simulink model "pendulam"  (R2019a)
settings: Solver=VariableStepAuto  StartTime=0.0  StopTime=10  FixedStep=0.01  MaxStep=0.05  MinStep=0.001  RelTol=1e-3
undefined symbols (not defined in the file): sigbuilder_block
settings Model: Creator=HPP  LastModifiedBy=vardhah
settings SolverCC: InitialStep=0.01
settings DebuggingCC: UnderSpecifiedDimensionMsg=warning

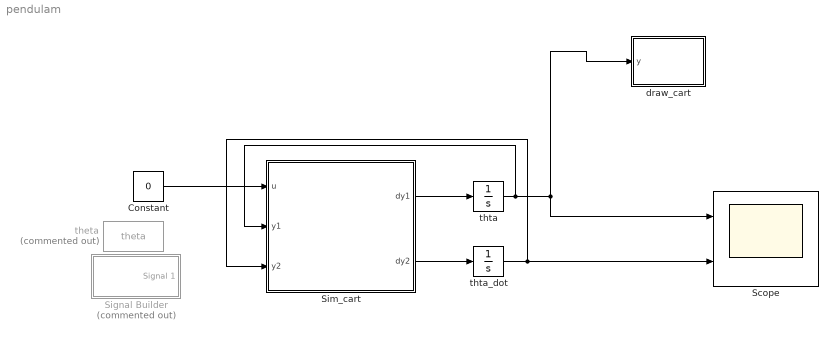
== system pendulam ==
  Constant : Constant  Value=0
  Scope : Scope  NumInputPorts=2
  Signal Builder : Subsystem  Tag=STV Subsys  Commented=on  LoadFcn=sigbuilder_block('load');  StartFcn=sigbuilder_block('start');  StopFcn=sigbuilder_block('stop');  ClipboardFcn=sigbuilder_block('clipboard');  mask(Sigbuilder block){tuvar=[0:10]}
      mask help: Simulink:masks:SigbuilderBlock_MD
      mask init:
      | if ~strcmp(get_param(bdroot(gcbh),'SimulationStatus'),'stopped') tuvar = sigbuilder_block('maskInit'); end
      settings: CopyFcn=sigbuilder_block('copy');  DeleteFcn=sigbuilder_block('delete');  ModelCloseFcn=sigbuilder_block('modelClose');  PreSaveFcn=sigbuilder_block('preSave');  PauseFcn=sigbuilder_block('pause');  ContinueFcn=sigbuilder_block('continue');  NameChangeFcn=sigbuilder_block('namechange');  OpenFcn=sigbuilder_block('open',[437.6 199.2 550.4 400 ]);  CloseFcn=sigbuilder_block('close');
      mask Display: plot(0, 0, 100, 100,[2, 2, 32, 32, 2], [68, 8, 8, 68, 68],[32, 2], [38, 38], [32, 19, 2],[53, 60, 44], [32, 17, 17, 2],[16, 16, 31, 31]);txt = getActiveGroup(gcbh);text(2, 100, txt,'verticalAlignment', 'top');
  Sim_cart : MATLAB Function  TreatAsAtomicUnit=on
  draw_cart : MATLAB Function  TreatAsAtomicUnit=on
  theta : ToWorkspace  Commented=on  VariableName=theta  SaveFormat=Timeseries  SampleTime=-1
  thta : Integrator  InitialCondition=pi/2
  thta_dot : Integrator
  wires:
  Sim_cart/1(dy1) -> thta/1
  Sim_cart/2(dy2) -> thta_dot/1
  thta_dot/1 -> Sim_cart/3(y2), Scope/2
  Constant/1 -> Sim_cart/1(u)
  thta/1 -> Sim_cart/2(y1), draw_cart/1(y), Scope/1

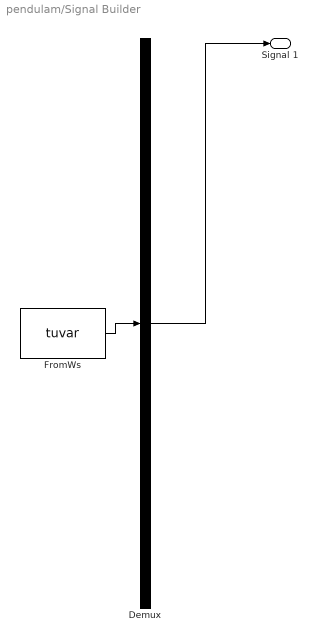
== system pendulam/Signal Builder ==
  Demux : Demux  Tag=STV Demux  Outputs=1
  FromWs : FromWorkspace  Tag=STV FromWs  VariableName=tuvar  SampleTime=0
      SigBuilderData=|
      | common.afterFinalStr = 'Extrapolate'
      | common.sampleTime = 0
      | dataSet.timeRange = [0 10]
      | dataSet.name = 'Group 1'
      | sbobj.Groups.Name = 'Group 1'
      | sbobj.Groups.Signals.Name = 'Signal 1'
      | sbobj.Groups.Signals.XData = [0 4 4 6 6 10]
      | sbobj.Groups.Signals.YData = [0 0 1 1 0 0]
  Signal 1 : Outport  Tag=STV Outport
  wires:
  Demux/1 -> Signal 1/1
  FromWs/1 -> Demux/1

== matlab function pendulam/draw_cart ==
  data: y input
function drawcartpend(y)
x = y;

m = 1;
L = 2;

O=[0 0];
axis(gca,'equal');
axis([-0.7 0.7 -0.7 0.2]);

%mass point
P=L*[sin(x) -cos(x)];
%circle in origin
O_circ=viscircles(O,0.01);
%pendulam 
pend=line([O(1) P(1)],[O(2) P(2)]);
%Ball
ball=viscircles(P,0.05);




% kinematics
% x = 3;        % cart position
% th = 3*pi/2;   % pendulum angle

% dimensions
% L = 2;  % pendulum length
W = 1*sqrt(M/5);  % cart width
H = .5*sqrt(M/5); % cart height
wr = .2; % wheel radius
mr = .3*sqrt(m); % mass radius

% positions
% y = wr/2; % cart vertical position
y = wr/2+H/2; % cart vertical position
w1x = x-.9*W/2;
w1y = 0;
w2x = x+.9*W/2-wr;
w2y = 0;

px = x + L*sin(th);
py = y - L*cos(th);

plot([-10 10],[0 0],'k','LineWidth',2)
hold on
rectangle('Position',[x-W/2,y-H/2,W,H],'Curvature',.1,'FaceColor',[1 0.1 0.1])
rectangle('Position',[w1x,w1y,wr,wr],'Curvature',1,'FaceColor',[0 0 0])
rectangle('Position',[w2x,w2y,wr,wr],'Curvature',1,'FaceColor',[0 0 0])

plot([x px],[y py],'k','LineWidth',2)

rectangle('Position',[px-mr/2,py-mr/2,mr,mr],'Curvature',1,'FaceColor',[.1 0.1 1])

% set(gca,'YTick',[])
% set(gca,'XTick',[])
xlim([-10 10]);
ylim([-2 2.5]);
%set(gcf,'Position',[100 550 500 400])
% box off
drawnow
hold off

== matlab function pendulam/Sim_cart ==
  settings: updateMethod=DISCRETE
  data: u input; y1 input; dy1 output size=1; dy2 output size=1; y2 input
function [dy1,dy2] = pend(u,y1,y2)

m = 1;
L = 2;
g = 10;
b = 5;

Sy = sin(y1);
D = m*L*L;

dy1 = y2;
dy2 = (1/D)*(-m*g*L*Sy - b*y2) +(1/D)*u;
end
